simulink model "Snapbot_4_leg"  (R2019b)
settings: Solver=FixedStepAuto  StartTime=0.0  StopTime=10  FixedStep=0.001  RelTol=1e-3
PreLoadFcn:
  | startup_Contact_Forces;
InitFcn:
  | SnapbotParameters;
StopFcn:
  | plot3(out.simout.data(:,1),out.simout.data(:,2),out.simout.data(:,3))
  | hold on;
  | plot3(out.simout.data(:,4),out.simout.data(:,5),out.simout.data(:,6))
  | plot3(out.simout.data(:,7),out.simout.data(:,8),out.simout.data(:,9))
  | plot3(out.simout.data(:,10),out.simout.data(:,11),out.simout.data(:,12))
  | grid on
  | grid minor
  | axis square
  | 
  | view(2)
model workspace (MATLAB code in the model file):
  | % Simscape(TM) Multibody(TM) version: 7.0
  | 
  | % This is a model data file derived from a Simscape Multibody Import XML file using the smimport function.
  | % The data in this file sets the block parameter values in an imported Simscape Multibody model.
  | % For more information on this file, see the smimport function help page in the Simscape Multibody documentation.
  | % You can modify numerical values, but avoid any other changes to this file.
  | % Do not add code to this file. Do not edit the physical units shown in comments.
  | 
  | %%%VariableName:smiData
  | 
  | 
  | %============= RigidTransform =============%
  | 
  | %Initialize the RigidTransform structure array by filling in null values.
  | smiData.RigidTransform(34).translation = [0.0 0.0 0.0];
  | smiData.RigidTransform(34).angle = 0.0;
  | smiData.RigidTransform(34).axis = [0.0 0.0 0.0];
  | smiData.RigidTransform(34).ID = '';
  | 
  | %Translation Method - Cartesian
  | %Rotation Method - Arbitrary Axis
  | smiData.RigidTransform(1).translation = [0 0 3.5000000000000031];  % mm
  | smiData.RigidTransform(1).angle = 0;  % rad
  | smiData.RigidTransform(1).axis = [0 0 0];
  | smiData.RigidTransform(1).ID = 'B[Leg_Assembly_Y-P:Leg_part_01_yaw-1:-:Leg_Assembly_Y-P:v4_Hyb_X-430_IDLE_uncut-1]';
  | 
  | %Translation Method - Cartesian
  | %Rotation Method - Arbitrary Axis
  | smiData.RigidTransform(2).translation = [-1.7352785874891197e-13 -35.250000000000064 1.6342482922482304e-13];  % mm
  | smiData.RigidTransform(2).angle = 3.1415926535897931;  % rad
  | smiData.RigidTransform(2).axis = [0 0.70710678118654746 0.70710678118654757];
  | smiData.RigidTransform(2).ID = 'F[Leg_Assembly_Y-P:Leg_part_01_yaw-1:-:Leg_Assembly_Y-P:v4_Hyb_X-430_IDLE_uncut-1]';
  | 
  | %Translation Method - Cartesian
  | %Rotation Method - Arbitrary Axis
  | smiData.RigidTransform(3).translation = [18.999999999999989 0 -21.500000000000018];  % mm
  | smiData.RigidTransform(3).angle = 2.0943951023931957;  % rad
  | smiData.RigidTransform(3).axis = [0.57735026918962562 0.57735026918962584 0.57735026918962584];
  | smiData.RigidTransform(3).ID = 'B[Leg_Assembly_Y-P:Leg_part_02_Yaw-1:-:Leg_Assembly_Y-P:v4_Hyb_X-430_IDLE_uncut-1]';
  | 
  | %Translation Method - Cartesian
  | %Rotation Method - Arbitrary Axis
  | smiData.RigidTransform(4).translation = [-1.5265566588595902e-12 -1.2221335055073723e-12 19.000000000000597];  % mm
  | smiData.RigidTransform(4).angle = 4.7102773760513257e-16;  % rad
  | smiData.RigidTransform(4).axis = [7.8504622934188734e-17 1 1.8488927466117461e-32];
  | smiData.RigidTransform(4).ID = 'F[Leg_Assembly_Y-P:Leg_part_02_Yaw-1:-:Leg_Assembly_Y-P:v4_Hyb_X-430_IDLE_uncut-1]';
  | 
  | %Translation Method - Cartesian
  | %Rotation Method - Arbitrary Axis
  | smiData.RigidTransform(5).translation = [8.3000000000000025 6 -1.5000000000000013];  % mm
  | smiData.RigidTransform(5).angle = 3.1415926535897931;  % rad
  | smiData.RigidTransform(5).axis = [1 0 0];
  | smiData.RigidTransform(5).ID = 'B[Leg_Assembly_Y-P:Leg_part_02_Yaw-1:-:Leg_Assembly_Y-P:v4_Hyb_X-430_IDLE_uncut-2]';
  | 
  | %Translation Method - Cartesian
  | %Rotation Method - Arbitrary Axis
  | smiData.RigidTransform(6).translation = [-8.0000000000000178 -36.75000000000005 6.0000000000000284];  % mm
  | smiData.RigidTransform(6).angle = 3.1415926535897931;  % rad
  | smiData.RigidTransform(6).axis = [-0 0.70710678118654757 -0.70710678118654746];
  | smiData.RigidTransform(6).ID = 'F[Leg_Assembly_Y-P:Leg_part_02_Yaw-1:-:Leg_Assembly_Y-P:v4_Hyb_X-430_IDLE_uncut-2]';
  | 
  | %Translation Method - Cartesian
  | %Rotation Method - Arbitrary Axis
  | smiData.RigidTransform(7).translation = [-5.7500000000000053 17.750000000000004 20.999999999999993];  % mm
  | smiData.RigidTransform(7).angle = 2.0943951023931953;  % rad
  | smiData.RigidTransform(7).axis = [0.57735026918962584 -0.57735026918962584 0.57735026918962584];
  | smiData.RigidTransform(7).ID = 'B[Leg_Assembly_Y-P:Leg_part_03-1:-:Leg_Assembly_Y-P:v4_Hyb_X-430_IDLE_uncut-2]';
  | 
  | %Translation Method - Cartesian
  | %Rotation Method - Arbitrary Axis
  | smiData.RigidTransform(8).translation = [-17.749999999998572 -3.9999999999999183 5.9999999999999556];  % mm
  | smiData.RigidTransform(8).angle = 2.0943951023931953;  % rad
  | smiData.RigidTransform(8).axis = [0.57735026918962584 0.57735026918962584 0.57735026918962584];
  | smiData.RigidTransform(8).ID = 'F[Leg_Assembly_Y-P:Leg_part_03-1:-:Leg_Assembly_Y-P:v4_Hyb_X-430_IDLE_uncut-2]';
  | 
  | %Translation Method - Cartesian
  | %Rotation Method - Arbitrary Axis
  | smiData.RigidTransform(9).translation = [48 0 0];  % mm
  | smiData.RigidTransform(9).angle = 2.0943951023931953;  % rad
  | smiData.RigidTransform(9).axis = [-0.57735026918962584 -0.57735026918962584 0.57735026918962584];
  | smiData.RigidTransform(9).ID = 'B[Leg_Assembly_Y-P:Leg_part_04-1:-:Leg_Assembly_Y-P:v4_Hyb_X-430_IDLE_uncut-2]';
  | 
  | %Translation Method - Cartesian
  | %Rotation Method - Arbitrary Axis
  | smiData.RigidTransform(10).translation = [-1.8746248997558723e-10 -7.7324813219092903e-12 24.00000000000599];  % mm
  | smiData.RigidTransform(10).angle = 3.1415926535897927;  % rad
  | smiData.RigidTransform(10).axis = [-1 -5.392603844284259e-33 2.7755575615628907e-17];
  | smiData.RigidTransform(10).ID = 'F[Leg_Assembly_Y-P:Leg_part_04-1:-:Leg_Assembly_Y-P:v4_Hyb_X-430_IDLE_uncut-2]';
  | 
  | %Translation Method - Cartesian
  | %Rotation Method - Arbitrary Axis
  | smiData.RigidTransform(11).translation = [21.999999999999993 6.0000000000000124 -15.000000000000009];  % mm
  | smiData.RigidTransform(11).angle = 0;  % rad
  | smiData.RigidTransform(11).axis = [0 0 0];
  | smiData.RigidTransform(11).ID = 'B[Leg_Assembly_Y-P:Leg_part_03-1:-:Leg_Assembly_Y-P:Leg_part_06-1]';
  | 
  | %Translation Method - Cartesian
  | %Rotation Method - Arbitrary Axis
  | smiData.RigidTransform(12).translation = [-25.499999999999105 -3.2214586553891422e-10 -47.43000000032751];  % mm
  | smiData.RigidTransform(12).angle = 2.0943951023931828;  % rad
  | smiData.RigidTransform(12).axis = [0.5773502691896234 0.57735026918962151 0.57735026918963239];
  | smiData.RigidTransform(12).ID = 'F[Leg_Assembly_Y-P:Leg_part_03-1:-:Leg_Assembly_Y-P:Leg_part_06-1]';
  | 
  | %Translation Method - Cartesian
  | %Rotation Method - Arbitrary Axis
  | smiData.RigidTransform(13).translation = [18.500000000000004 0 0];  % mm
  | smiData.RigidTransform(13).angle = 2.0943951023931957;  % rad
  | smiData.RigidTransform(13).axis = [-0.57735026918962584 -0.57735026918962573 0.57735026918962573];
  | smiData.RigidTransform(13).ID = 'B[Leg_Assembly_Y-P:Leg_part_05-1:-:Leg_Assembly_Y-P:Leg_part_04-1]';
  | 
  | %Translation Method - Cartesian
  | %Rotation Method - Arbitrary Axis
  | smiData.RigidTransform(14).translation = [5.4999999999949978 -8.3794303905713249e-10 -60.000000000037232];  % mm
  | smiData.RigidTransform(14).angle = 2.0943951023931917;  % rad
  | smiData.RigidTransform(14).axis = [0.57735026918961896 0.57735026918962451 0.57735026918963384];
  | smiData.RigidTransform(14).ID = 'F[Leg_Assembly_Y-P:Leg_part_05-1:-:Leg_Assembly_Y-P:Leg_part_04-1]';
  | 
  | %Translation Method - Cartesian
  | %Rotation Method - Arbitrary Axis
  | smiData.RigidTransform(15).translation = [-4.5000000000000009 25.000000000000004 0];  % mm
  | smiData.RigidTransform(15).angle = 2.0943951023931953;  % rad
  | smiData.RigidTransform(15).axis = [-0.57735026918962584 -0.57735026918962584 0.57735026918962584];
  | smiData.RigidTransform(15).ID = 'B[Leg_Assembly_Y-P:Leg_part_05-1:-:Leg_Assembly_Y-P:Leg_part_06-1]';
  | 
  | %Translation Method - Cartesian
  | %Rotation Method - Arbitrary Axis
  | smiData.RigidTransform(16).translation = [9.0000000000012914 1.0276604186564152e-10 7.8563660354995227e-11];  % mm
  | smiData.RigidTransform(16).angle = 2.0943951023931957;  % rad
  | smiData.RigidTransform(16).axis = [0.57735026918962573 0.57735026918962595 0.57735026918962562];
  | smiData.RigidTransform(16).ID = 'F[Leg_Assembly_Y-P:Leg_part_05-1:-:Leg_Assembly_Y-P:Leg_part_06-1]';
  | 
  | %Translation Method - Cartesian
  | %Rotation Method - Arbitrary Axis
  | smiData.RigidTransform(17).translation = [-29.148138792437695 31.324765133364561 -50.486057334570788];  % mm
  | smiData.RigidTransform(17).angle = 0.85969556486762955;  % rad
  | smiData.RigidTransform(17).axis = [-0.88342402684813537 0.43430848851138693 -0.17589236934665334];
  | smiData.RigidTransform(17).ID = 'B[Body_Frame-2:-:cover_IMU-1]';
  | 
  | %Translation Method - Cartesian
  | %Rotation Method - Arbitrary Axis
  | smiData.RigidTransform(18).translation = [-29.14813879243771 -3.6752348666354493 -50.486057334570788];  % mm
  | smiData.RigidTransform(18).angle = 0.85969556486762955;  % rad
  | smiData.RigidTransform(18).axis = [-0.88342402684813537 0.43430848851138693 -0.17589236934665334];
  | smiData.RigidTransform(18).ID = 'F[Body_Frame-2:-:cover_IMU-1]';
  | 
  | %Translation Method - Cartesian
  | %Rotation Method - Arbitrary Axis
  | smiData.RigidTransform(19).translation = [-17.98437038909324 16.010419740604625 -58.898751217406286];  % mm
  | smiData.RigidTransform(19).angle = 2.5668813081404753;  % rad
  | smiData.RigidTransform(19).axis = [-0.54469904781872214 -0.67552162020226258 0.49696427230203144];
  | smiData.RigidTransform(19).ID = 'B[Body_Frame-2:-:Leg_Assembly_Y-P-4:Leg_part_01_yaw-1]';
  | 
  | %Translation Method - Cartesian
  | %Rotation Method - Arbitrary Axis
  | smiData.RigidTransform(20).translation = [-13.874453980679554 8.010419740604668 -21.000000000000121];  % mm
  | smiData.RigidTransform(20).angle = 1.5933089052267591;  % rad
  | smiData.RigidTransform(20).axis = [0.454741574326607 0.14837486987204307 0.87817708838787945];
  | smiData.RigidTransform(20).ID = 'F[Body_Frame-2:-:Leg_Assembly_Y-P-4:Leg_part_01_yaw-1]';
  | 
  | %Translation Method - Cartesian
  | %Rotation Method - Arbitrary Axis
  | smiData.RigidTransform(21).translation = [29.999999999999968 24.020839481209347 -51.961524227066349];  % mm
  | smiData.RigidTransform(21).angle = 2.3875525638501713;  % rad
  | smiData.RigidTransform(21).axis = [0.97769691900991618 0.078837114487629617 0.19466238449629056];
  | smiData.RigidTransform(21).ID = 'B[Body_Frame-2:-:Leg_Assembly_Y-P-3:Leg_part_01_yaw-1]';
  | 
  | %Translation Method - Cartesian
  | %Rotation Method - Arbitrary Axis
  | smiData.RigidTransform(22).translation = [-2.6467716907063732e-13 16.020839481209734 -21.000000000000327];  % mm
  | smiData.RigidTransform(22).angle = 2.8078721686781996;  % rad
  | smiData.RigidTransform(22).axis = [0.061302152168851563 -0.3413768904692025 0.9379252980877768];
  | smiData.RigidTransform(22).ID = 'F[Body_Frame-2:-:Leg_Assembly_Y-P-3:Leg_part_01_yaw-1]';
  | 
  | %Translation Method - Cartesian
  | %Rotation Method - Arbitrary Axis
  | smiData.RigidTransform(23).translation = [30.000000000000529 24.020839481209347 51.961524227066029];  % mm
  | smiData.RigidTransform(23).angle = 0.85969556486763532;  % rad
  | smiData.RigidTransform(23).axis = [0.88342402684813182 0.43430848851139281 0.17589236934665636];
  | smiData.RigidTransform(23).ID = 'B[Body_Frame-2:-:Leg_Assembly_Y-P-2:Leg_part_01_yaw-1]';
  | 
  | %Translation Method - Cartesian
  | %Rotation Method - Arbitrary Axis
  | smiData.RigidTransform(24).translation = [3.3395508580724709e-13 16.020839481209283 -21.000000000000096];  % mm
  | smiData.RigidTransform(24).angle = 0.78005530127659528;  % rad
  | smiData.RigidTransform(24).axis = [0.88538441591606198 -0.1589913427291928 0.43682512403723089];
  | smiData.RigidTransform(24).ID = 'F[Body_Frame-2:-:Leg_Assembly_Y-P-2:Leg_part_01_yaw-1]';
  | 
  | %Translation Method - Cartesian
  | %Rotation Method - Arbitrary Axis
  | smiData.RigidTransform(25).translation = [0 16.0208394812094 -21.000000000000004];  % mm
  | smiData.RigidTransform(25).angle = 2.4434609527920594;  % rad
  | smiData.RigidTransform(25).axis = [-1 -2.4245288061633076e-16 6.6613381477509383e-16];
  | smiData.RigidTransform(25).ID = 'B[Leg_Assembly_Y-P-1:Leg_part_01_yaw-1:-:Body_Frame-2]';
  | 
  | %Translation Method - Cartesian
  | %Rotation Method - Arbitrary Axis
  | smiData.RigidTransform(26).translation = [-29.999999999999616 24.020839481209507 51.961524227066668];  % mm
  | smiData.RigidTransform(26).angle = 2.4682098215588222;  % rad
  | smiData.RigidTransform(26).axis = [-0.96166828182989783 -0.093787209197190524 -0.25767823950294055];
  | smiData.RigidTransform(26).ID = 'F[Leg_Assembly_Y-P-1:Leg_part_01_yaw-1:-:Body_Frame-2]';
  | 
  | %Translation Method - Cartesian
  | %Rotation Method - Arbitrary Axis
  | smiData.RigidTransform(27).translation = [58.296277584874822 -3.6752348666354502 0];  % mm
  | smiData.RigidTransform(27).angle = 1.750366012803156;  % rad
  | smiData.RigidTransform(27).axis = [0.83481712947898612 0.38928162063502708 0.38928162063502636];
  | smiData.RigidTransform(27).ID = 'B[cover-2:-:Body_Frame-2]';
  | 
  | %Translation Method - Cartesian
  | %Rotation Method - Arbitrary Axis
  | smiData.RigidTransform(28).translation = [-58.29627758487473 -15.324765133364487 1.1215639593173864e-12];  % mm
  | smiData.RigidTransform(28).angle = 2.5346467848844099;  % rad
  | smiData.RigidTransform(28).axis = [0.31314561301496879 -0.67154293423781619 -0.67154293423782185];
  | smiData.RigidTransform(28).ID = 'F[cover-2:-:Body_Frame-2]';
  | 
  | %Translation Method - Cartesian
  | %Rotation Method - Arbitrary Axis
  | smiData.RigidTransform(29).translation = [-0.53570167355018738 37.318511693782625 54.569829435763872];  % mm
  | smiData.RigidTransform(29).angle = 0;  % rad
  | smiData.RigidTransform(29).axis = [0 0 0];
  | smiData.RigidTransform(29).ID = 'AssemblyGround[Leg_Assembly_Y-P-1:Leg_part_01_yaw-1]';
  | 
  | %Translation Method - Cartesian
  | %Rotation Method - Arbitrary Axis
  | smiData.RigidTransform(30).translation = [-0.53570167355018394 37.318511693782625 54.569829435763872];  % mm
  | smiData.RigidTransform(30).angle = 0;  % rad
  | smiData.RigidTransform(30).axis = [0 0 0];
  | smiData.RigidTransform(30).ID = 'AssemblyGround[Leg_Assembly_Y-P-3:Leg_part_01_yaw-1]';
  | 
  | %Translation Method - Cartesian
  | %Rotation Method - Arbitrary Axis
  | smiData.RigidTransform(31).translation = [-0.53570167355018217 37.318511693782625 54.56982943576385];  % mm
  | smiData.RigidTransform(31).angle = 0;  % rad
  | smiData.RigidTransform(31).axis = [0 0 0];
  | smiData.RigidTransform(31).ID = 'AssemblyGround[Leg_Assembly_Y-P-4:Leg_part_01_yaw-1]';
  | 
  | %Translation Method - Cartesian
  | %Rotation Method - Arbitrary Axis
  | smiData.RigidTransform(32).translation = [-0.53570167355018561 37.318511693782625 54.569829435763886];  % mm
  | smiData.RigidTransform(32).angle = 0;  % rad
  | smiData.RigidTransform(32).axis = [0 0 0];
  | smiData.RigidTransform(32).ID = 'AssemblyGround[Leg_Assembly_Y-P-2:Leg_part_01_yaw-1]';
  | 
  | %Translation Method - Cartesian
  | %Rotation Method - Arbitrary Axis
  | smiData.RigidTransform(33).translation = [16.947427364988048 -132.5 -0.35447398452139084];  % mm
  | smiData.RigidTransform(33).angle = 0;  % rad
  | smiData.RigidTransform(33).axis = [0 0 0];
  | smiData.RigidTransform(33).ID = 'RootGround[floor-1]';
  | 
  | %Translation Method - Cartesian
  | %Rotation Method - Arbitrary Axis
  | smiData.RigidTransform(34).translation = [2.4083582801206584 -17.449369734884318 -0.97062236223489184];  % mm
  | smiData.RigidTransform(34).angle = 3.1415926535897927;  % rad
  | smiData.RigidTransform(34).axis = [-1.8561360843499775e-09 2.3245294513264802e-16 1];
  | smiData.RigidTransform(34).ID = 'SixDofRigidTransform[cover-2]';
  | 
  | 
  | %============= Solid =============%
  | %Center of Mass (CoM) %Moments of Inertia (MoI) %Product of Inertia (PoI)
  | 
  | %Initialize the Solid structure array by filling in null values.
  | smiData.Solid(11).mass = 0.0;
  | smiData.Solid(11).CoM = [0.0 0.0 0.0];
  | smiData.Solid(11).MoI = [0.0 0.0 0.0];
  | smiData.Solid(11).PoI = [0.0 0.0 0.0];
  | smiData.Solid(11).color = [0.0 0.0 0.0];
  | smiData.Solid(11).opacity = 0.0;
  | smiData.Solid(11).ID = '';
  | 
  | %Inertia Type - Custom
  | %Visual Properties - Simple
  | smiData.Solid(1).mass = 0.011859040673008397;  % kg
  | smiData.Solid(1).CoM = [9.2568952005630604e-05 1.191765890643393 -6.4265217754949023e-05];  % mm
  | smiData.Solid(1).MoI = [12.336903139260382 24.543407766477525 12.336924066027152];  % kg*mm^2
  | smiData.Solid(1).PoI = [1.0093449377553896e-06 3.0788090295607977e-05 -1.064469578641841e-06];  % kg*mm^2
  | smiData.Solid(1).color = [0.792156862745098 0.81960784313725488 0.93333333333333335];
  | smiData.Solid(1).opacity = 1;
  | smiData.Solid(1).ID = 'cover*:*Default';
  | 
  | %Inertia Type - Custom
  | %Visual Properties - Simple
  | smiData.Solid(2).mass = 0.012023631787858334;  % kg
  | smiData.Solid(2).CoM = [-0.29734349259876186 1.2054189328895923 0.00017861160100909334];  % mm
  | smiData.Solid(2).MoI = [12.313344376366921 24.562977425030333 12.378785765398183];  % kg*mm^2
  | smiData.Solid(2).PoI = [1.0647394470527272e-05 -8.7602005901832794e-05 0.00062815776109033676];  % kg*mm^2
  | smiData.Solid(2).color = [0.792156862745098 0.81960784313725488 0.93333333333333335];
  | smiData.Solid(2).opacity = 1;
  | smiData.Solid(2).ID = 'cover_IMU*:*Default';
  | 
  | %Inertia Type - Custom
  | %Visual Properties - Simple
  | smiData.Solid(3).mass = 0.01532092516699415;  % kg
  | smiData.Solid(3).CoM = [23.99999768920209 1.296167806282416 -35.100094443023529];  % mm
  | smiData.Solid(3).MoI = [10.22123294031608 14.203511884952171 5.0157635391797406];  % kg*mm^2
  | smiData.Solid(3).PoI = [0.58071119483444822 9.2473756106630214e-07 -5.4914041407852197e-06];  % kg*mm^2
  | smiData.Solid(3).color = [1 0.38823529411764707 0.41960784313725491];
  | smiData.Solid(3).opacity = 1;
  | smiData.Solid(3).ID = 'Leg_part_04*:*Default';
  | 
  | %Inertia Type - Custom
  | %Visual Properties - Simple
  | smiData.Solid(4).mass = 0.022715083434313929;  % kg
  | smiData.Solid(4).CoM = [4.7495790017590746e-05 -5.291488289899466e-07 0.51650579217012571];  % mm
  | smiData.Solid(4).MoI = [6.0201227624572118 7.3567997591054697 10.813457729002581];  % kg*mm^2
  | smiData.Solid(4).PoI = [5.9445977678909571e-08 -2.8721317733849146e-06 -2.6844578170485016e-06];  % kg*mm^2
  | smiData.Solid(4).color = [0.027450980392156862 1 0.027450980392156862];
  | smiData.Solid(4).opacity = 1;
  | smiData.Solid(4).ID = 'Leg_part_02_Yaw*:*Default';
  | 
  | %Inertia Type - Custom
  | %Visual Properties - Simple
  | smiData.Solid(5).mass = 0.0061788723822202912;  % kg
  | smiData.Solid(5).CoM = [4.2543802409912486 -4.6300920972242539 -20.149819352752832];  % mm
  | smiData.Solid(5).MoI = [2.2893274182864185 2.0053458866812135 0.35993641872183124];  % kg*mm^2
  | smiData.Solid(5).PoI = [0.20173149787382891 -0.0054107076234519375 0.0070268738351532264];  % kg*mm^2
  | smiData.Solid(5).color = [0.8666666666666667 0.46666666666666667 0.094117647058823528];
  | smiData.Solid(5).opacity = 1;
  | smiData.Solid(5).ID = 'Leg_part_06*:*Default';
  | 
  | %Inertia Type - Custom
  | %Visual Properties - Simple
  | smiData.Solid(6).mass = 0.022008322051922567;  % kg
  | smiData.Solid(6).CoM = [-0.00020078562164607593 -0.086645709821882896 -7.0226871847428294];  % mm
  | smiData.Solid(6).MoI = [6.5441760223709844 5.812065440337185 5.5882327823375331];  % kg*mm^2
  | smiData.Solid(6).PoI = [-0.022603449848343178 -3.3526868327938216e-05 -5.8881839764321484e-05];  % kg*mm^2
  | smiData.Solid(6).color = [0.9882352941176471 0.73725490196078436 0.51764705882352935];
  | smiData.Solid(6).opacity = 1;
  | smiData.Solid(6).ID = 'Leg_part_01_yaw*:*Default';
  | 
  | %Inertia Type - Custom
  | %Visual Properties - Simple
  | smiData.Solid(7).mass = 0.015928924279537775;  % kg
  | smiData.Solid(7).CoM = [5.5724533955433548 0.60923661115773253 14.965495324586268];  % mm
  | smiData.Solid(7).MoI = [6.7178267454302487 3.3961346093070595 5.3516535264104625];  % kg*mm^2
  | smiData.Solid(7).PoI = [0.0029589860947701109 0.0090414356066351384 -0.14024072638650095];  % kg*mm^2
  | smiData.Solid(7).color = [0.50196078431372548 1 1];
  | smiData.Solid(7).opacity = 1;
  | smiData.Solid(7).ID = 'Leg_part_03*:*Default';
  | 
  | %Inertia Type - Custom
  | %Visual Properties - Simple
  | smiData.Solid(8).mass = 0.014765646142892601;  % kg
  | smiData.Solid(8).CoM = [1.2086758180566385e-05 38.516029865216893 1.6102137949923504e-05];  % mm
  | smiData.Solid(8).MoI = [11.438112427079185 0.88080259805912409 11.92628093115035];  % kg*mm^2
  | smiData.Solid(8).PoI = [1.3310978325613474e-06 5.7966270338224739e-06 1.0118234092923484e-06];  % kg*mm^2
  | smiData.Solid(8).color = [0.039215686274509803 0.63137254901960782 0.90588235294117647];
  | smiData.Solid(8).opacity = 1;
  | smiData.Solid(8).ID = 'Leg_part_05*:*Default';
  | 
  | %Inertia Type - Custom
  | %Visual Properties - Simple
  | smiData.Solid(9).mass = 0.043283962506312147;  % kg
  | smiData.Solid(9).CoM = [0 -11.629154441205351 0.58622657822569424];  % mm
  | smiData.Solid(9).MoI = [11.945660403890638 6.9373449472329343 10.473897647404554];  % kg*mm^2
  | smiData.Solid(9).PoI = [-0.010479195470367004 0 0];  % kg*mm^2
  | smiData.Solid(9).color = [0.50196078431372548 0.50196078431372548 0.50196078431372548];
  | smiData.Solid(9).opacity = 1;
  | smiData.Solid(9).ID = 'v4_Hyb_X-430_IDLE_uncut*:*Default';
  | 
  | %Inertia Type - Custom
  | %Visual Properties - Simple
  | smiData.Solid(10).mass = 0.06914285683427808;  % kg
  | smiData.Solid(10).CoM = [-6.5363881170266666e-08 8.0286872966298493 -0.84505300940729655];  % mm
  | smiData.Solid(10).MoI = [133.83817269769423 248.31514966138266 134.30804068565411];  % kg*mm^2
  | smiData.Solid(10).PoI = [0.10611953301327913 3.6362610588971529e-07 -3.5551675916145607e-07];  % kg*mm^2
  | smiData.Solid(10).color = [0.75294117647058822 0.75294117647058822 0.75294117647058822];
  | smiData.Solid(10).opacity = 1;
  | smiData.Solid(10).ID = 'Body_Frame*:*Default';
  | 
  | %Inertia Type - Custom
  | %Visual Properties - Simple
  | smiData.Solid(11).mass = 49.999999999999993;  % kg
  | smiData.Solid(11).CoM = [0 25.000000000000004 0];  % mm
  | smiData.Solid(11).MoI = [4177083.333333334 8333333.3333333358 4177083.333333333];  % kg*mm^2
  | smiData.Solid(11).PoI = [0 -7.6327832942979522e-10 0];  % kg*mm^2
  | smiData.Solid(11).color = [0.792156862745098 0.81960784313725488 0.93333333333333335];
  | smiData.Solid(11).opacity = 1;
  | smiData.Solid(11).ID = 'floor*:*Default';
  | 
  | 
  | %============= Joint =============%
  | %X Revolute Primitive (Rx) %Y Revolute Primitive (Ry) %Z Revolute Primitive (Rz)
  | %X Prismatic Primitive (Px) %Y Prismatic Primitive (Py) %Z Prismatic Primitive (Pz) %Spherical Primitive (S)
  | %Constant Velocity Primitive (CV) %Lead Screw Primitive (LS)
  | %Position Target (Pos)
  | 
  | %Initialize the CylindricalJoint structure array by filling in null values.
  | smiData.CylindricalJoint(4).Rz.Pos = 0.0;
  | smiData.CylindricalJoint(4).Pz.Pos = 0.0;
  | smiData.CylindricalJoint(4).ID = '';
  | 
  | %This joint has been chosen as a cut joint. Simscape Multibody treats cut joints as algebraic constraints to solve closed kinematic loops. The imported model does not use the state target data for this joint.
  | smiData.CylindricalJoint(1).Rz.Pos = -40.005411760834875;  % deg
  | smiData.CylindricalJoint(1).Pz.Pos = 0;  % mm
  | smiData.CylindricalJoint(1).ID = '[Leg_Assembly_Y-P-1:Leg_part_05-1:-:Leg_Assembly_Y-P-1:Leg_part_06-1]';
  | 
  | %This joint has been chosen as a cut joint. Simscape Multibody treats cut joints as algebraic constraints to solve closed kinematic loops. The imported model does not use the state target data for this joint.
  | smiData.CylindricalJoint(2).Rz.Pos = -40.005411760841149;  % deg
  | smiData.CylindricalJoint(2).Pz.Pos = 0;  % mm
  | smiData.CylindricalJoint(2).ID = '[Leg_Assembly_Y-P-3:Leg_part_05-1:-:Leg_Assembly_Y-P-3:Leg_part_06-1]';
  | 
  | %This joint has been chosen as a cut joint. Simscape Multibody treats cut joints as algebraic constraints to solve closed kinematic loops. The imported model does not use the state target data for this joint.
  | smiData.CylindricalJoint(3).Rz.Pos = -40.005411760676694;  % deg
  | smiData.CylindricalJoint(3).Pz.Pos = 0;  % mm
  | smiData.CylindricalJoint(3).ID = '[Leg_Assembly_Y-P-4:Leg_part_05-1:-:Leg_Assembly_Y-P-4:Leg_part_06-1]';
  | 
  | %This joint has been chosen as a cut joint. Simscape Multibody treats cut joints as algebraic constraints to solve closed kinematic loops. The imported model does not use the state target data for this joint.
  | smiData.CylindricalJoint(4).Rz.Pos = -40.00541176081142;  % deg
  | smiData.CylindricalJoint(4).Pz.Pos = 0;  % mm
  | smiData.CylindricalJoint(4).ID = '[Leg_Assembly_Y-P-2:Leg_part_05-1:-:Leg_Assembly_Y-P-2:Leg_part_06-1]';
  | 
  | 
  | %Initialize the RevoluteJoint structure array by filling in null values.
  | smiData.RevoluteJoint(20).Rz.Pos = 0.0;
  | smiData.RevoluteJoint(20).ID = '';
  | 
  | smiData.RevoluteJoint(1).Rz.Pos = 8.9959671327898853e-15;  % deg
  | smiData.RevoluteJoint(1).ID = '[Leg_Assembly_Y-P-1:Leg_part_02_Yaw-1:-:Leg_Assembly_Y-P-1:v4_Hyb_X-430_IDLE_uncut-1]';
  | 
  | smiData.RevoluteJoint(2).Rz.Pos = -90;  % deg
  | smiData.RevoluteJoint(2).ID = '[Leg_Assembly_Y-P-1:Leg_part_03-1:-:Leg_Assembly_Y-P-1:v4_Hyb_X-430_IDLE_uncut-2]';
  | 
  | smiData.RevoluteJoint(3).Rz.Pos = 180;  % deg
  | smiData.RevoluteJoint(3).ID = '[Leg_Assembly_Y-P-1:Leg_part_04-1:-:Leg_Assembly_Y-P-1:v4_Hyb_X-430_IDLE_uncut-2]';
  | 
  | smiData.RevoluteJoint(4).Rz.Pos = -130.80925683646444;  % deg
  | smiData.RevoluteJoint(4).ID = '[Leg_Assembly_Y-P-1:Leg_part_03-1:-:Leg_Assembly_Y-P-1:Leg_part_06-1]';
  | 
  | smiData.RevoluteJoint(5).Rz.Pos = -179.19615492437049;  % deg
  | smiData.RevoluteJoint(5).ID = '[Leg_Assembly_Y-P-1:Leg_part_05-1:-:Leg_Assembly_Y-P-1:Leg_part_04-1]';
  | 
  | smiData.RevoluteJoint(6).Rz.Pos = 9.6985521658607794e-11;  % deg
  | smiData.RevoluteJoint(6).ID = '[Leg_Assembly_Y-P-3:Leg_part_02_Yaw-1:-:Leg_Assembly_Y-P-3:v4_Hyb_X-430_IDLE_uncut-1]';
  | 
  | smiData.RevoluteJoint(7).Rz.Pos = -90.000000000000014;  % deg
  | smiData.RevoluteJoint(7).ID = '[Leg_Assembly_Y-P-3:Leg_part_03-1:-:Leg_Assembly_Y-P-3:v4_Hyb_X-430_IDLE_uncut-2]';
  | 
  | smiData.RevoluteJoint(8).Rz.Pos = -179.99999999998752;  % deg
  | smiData.RevoluteJoint(8).ID = '[Leg_Assembly_Y-P-3:Leg_part_04-1:-:Leg_Assembly_Y-P-3:v4_Hyb_X-430_IDLE_uncut-2]';
  | 
  | smiData.RevoluteJoint(9).Rz.Pos = -130.80925683643747;  % deg
  | smiData.RevoluteJoint(9).ID = '[Leg_Assembly_Y-P-3:Leg_part_03-1:-:Leg_Assembly_Y-P-3:Leg_part_06-1]';
  | 
  | smiData.RevoluteJoint(10).Rz.Pos = -179.19615492439118;  % deg
  | smiData.RevoluteJoint(10).ID = '[Leg_Assembly_Y-P-3:Leg_part_05-1:-:Leg_Assembly_Y-P-3:Leg_part_04-1]';
  | 
  | smiData.RevoluteJoint(11).Rz.Pos = 1.7991934265579774e-14;  % deg
  | smiData.RevoluteJoint(11).ID = '[Leg_Assembly_Y-P-4:Leg_part_02_Yaw-1:-:Leg_Assembly_Y-P-4:v4_Hyb_X-430_IDLE_uncut-1]';
  | 
  | smiData.RevoluteJoint(12).Rz.Pos = -90;  % deg
  | smiData.RevoluteJoint(12).ID = '[Leg_Assembly_Y-P-4:Leg_part_03-1:-:Leg_Assembly_Y-P-4:v4_Hyb_X-430_IDLE_uncut-2]';
  | 
  | smiData.RevoluteJoint(13).Rz.Pos = 179.99999999960033;  % deg
  | smiData.RevoluteJoint(13).ID = '[Leg_Assembly_Y-P-4:Leg_part_04-1:-:Leg_Assembly_Y-P-4:v4_Hyb_X-430_IDLE_uncut-2]';
  | 
  | smiData.RevoluteJoint(14).Rz.Pos = -130.80925683712383;  % deg
  | smiData.RevoluteJoint(14).ID = '[Leg_Assembly_Y-P-4:Leg_part_03-1:-:Leg_Assembly_Y-P-4:Leg_part_06-1]';
  | 
  | smiData.RevoluteJoint(15).Rz.Pos = -179.19615492395255;  % deg
  | smiData.RevoluteJoint(15).ID = '[Leg_Assembly_Y-P-4:Leg_part_05-1:-:Leg_Assembly_Y-P-4:Leg_part_04-1]';
  | 
  | smiData.RevoluteJoint(16).Rz.Pos = 8.9959671327898869e-15;  % deg
  | smiData.RevoluteJoint(16).ID = '[Leg_Assembly_Y-P-2:Leg_part_02_Yaw-1:-:Leg_Assembly_Y-P-2:v4_Hyb_X-430_IDLE_uncut-1]';
  | 
  | smiData.RevoluteJoint(17).Rz.Pos = -90;  % deg
  | smiData.RevoluteJoint(17).ID = '[Leg_Assembly_Y-P-2:Leg_part_03-1:-:Leg_Assembly_Y-P-2:v4_Hyb_X-430_IDLE_uncut-2]';
  | 
  | smiData.RevoluteJoint(18).Rz.Pos = 180;  % deg
  | smiData.RevoluteJoint(18).ID = '[Leg_Assembly_Y-P-2:Leg_part_04-1:-:Leg_Assembly_Y-P-2:v4_Hyb_X-430_IDLE_uncut-2]';
  | 
  | smiData.RevoluteJoint(19).Rz.Pos = -130.80925683656244;  % deg
  | smiData.RevoluteJoint(19).ID = '[Leg_Assembly_Y-P-2:Leg_part_03-1:-:Leg_Assembly_Y-P-2:Leg_part_06-1]';
  | 
  | smiData.RevoluteJoint(20).Rz.Pos = -179.19615492424902;  % deg
  | smiData.RevoluteJoint(20).ID = '[Leg_Assembly_Y-P-2:Leg_part_05-1:-:Leg_Assembly_Y-P-2:Leg_part_04-1]';
values from neighbouring files (symbols this model uses):
  mass_xm430 = 82    [SnapbotParameters.m]
undefined symbols (not defined in the file or in its folder): smiData, X, Y, Z
libraries: sm_lib x191, nesl_utility x28, Contact_Forces_Lib x10
(part 1 of 6)
settings Model: Creator=Kevin_Home  LastModifiedBy=Kevin_Home
settings ExplorerConfigSet: InternalSimMechanicsExplorerSettings="<ExplorerConfiguration><canonicalview>default</canonicalview><AnimationSetting><BasePlaybackSpeed>1.0</BasePlaybackSpeed><PlaybackSpeedFactor>1.0</PlaybackSpeedFactor></AnimationSetting><TilePanel><TileInfo><Tiles Columns=\"1\" Count=\"1\" Rows=\"1\"><Column Weight=\"1\"/><Row Weight=\"1\"/><Tile Height=\"1\" Width=\"1\" X=\"0\" Y=\"0\"/></Tiles></TileInfo><SceneInfo><SceneViewer><BGColor><R>0.60000002384185791</R><G>1</G><B>1</B></BGColor><Camera><DoPerspective>off</DoPerspective><Position><X>-217.246830094688079</X><Y>113.108474411831537</Y><Z>52.8872630286014385</Z></Position><Center><X>-0.902430327962377987</X><Y>0.229218017573074917</Y><Z>0.175732092976339516</Z></Center><Up><X>0.442868139606599265</X><Y>0.8918375727327299</Y><Z>-0.0921604838506315804</Z></Up><ViewLimDist>1</ViewLimDist><YLim>0.501072049732542601</YLim><XLim>0.806169253347468473</XLim></Camera></SceneViewer></SceneInfo></TilePanel><MechEditorPanel><Cameras/><GfxPanelCameraMap/><VideoCreator><PlaybackSpeedRatio>1.0</PlaybackSpeedRatio><FrameRate>30</FrameRate><VideoFormat>MPEG-4</VideoFormat><FrameSize>auto</FrameSize></VideoCreator></MechEditorPanel></ExplorerConfiguration>"

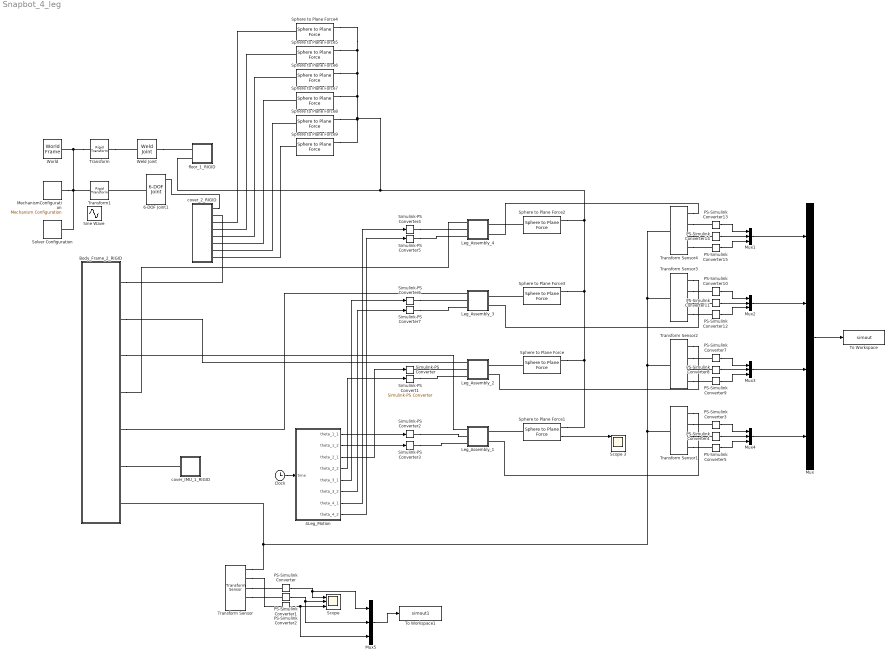
== system Snapbot_4_leg ==
  4Leg_Motion : MATLAB Function  TreatAsAtomicUnit=on
  6-DOF Joint1 : sm_lib/Joints/6-DOF Joint  JointMode=Normal  SenseConstraintForce=off  SenseConstraintForceX=off  SenseConstraintForceY=off  SenseConstraintForceZ=off  SenseConstraintTorque=off  SenseConstraintTorqueX=off  SenseConstraintTorqueY=off  SenseConstraintTorqueZ=off  SenseTotalForce=off  SenseTotalForceX=off  SenseTotalForceY=off  SenseTotalForceZ=off  SenseTotalTorque=off  SenseTotalTorqueX=off  SenseTotalTorqueY=off  SenseTotalTorqueZ=off  CompositeWrenchDir=FollowerOnBase  CompositeWrenchFrame=BaseFrame  PxEquilibriumPosition=0  PxEquilibriumPositionUnits=m  PxSpringStiffness=0  PxSpringStiffnessUnits=N/m  PxDampingCoefficient=0  PxDampingCoefficientUnits=N/(m/s)  PxTorqueActuationMode=NoTorque  PxMotionActuationMode=ComputedMotion  PxSensePosition=on  PxSenseVelocity=off  PxSenseAcceleration=off  PxSenseTorqueForce=off  PxSenseLowerLimitTorqueForce=off  PxSenseUpperLimitTorqueForce=off  PxLowerLimitSpecify=off  PxLowerLimitBound=-1  PxLowerLimitBoundUnits=m  PxLowerLimitStiffness=1e6  PxLowerLimitStiffnessUnits=N/m  PxLowerLimitDamping=1e3  PxLowerLimitDampingUnits=N/(m/s)  PxLowerLimitTransitionRegionWidth=1e-4  PxLowerLimitTransitionRegionWidthUnits=m  PxUpperLimitSpecify=off  PxUpperLimitBound=1  PxUpperLimitBoundUnits=m  PxUpperLimitStiffness=1e6  PxUpperLimitStiffnessUnits=N/m  PxUpperLimitDamping=1e3  PxUpperLimitDampingUnits=N/(m/s)  PxUpperLimitTransitionRegionWidth=1e-4  PxUpperLimitTransitionRegionWidthUnits=m  PxPositionTargetSpecify=off  PxPositionTargetPriority=High  PxPositionTargetValue=0  PxPositionTargetValueUnits=m  PxVelocityTargetSpecify=off  PxVelocityTargetPriority=High  PxVelocityTargetValue=0  PxVelocityTargetValueUnits=m/s  PyEquilibriumPosition=0  PyEquilibriumPositionUnits=m  PySpringStiffness=0  PySpringStiffnessUnits=N/m  PyDampingCoefficient=0  PyDampingCoefficientUnits=N/(m/s)  PyTorqueActuationMode=NoTorque  PyMotionActuationMode=ComputedMotion  PySensePosition=on  PySenseVelocity=off  PySenseAcceleration=off  PySenseTorqueForce=off  PySenseLowerLimitTorqueForce=off  PySenseUpperLimitTorqueForce=off  PyLowerLimitSpecify=off  PyLowerLimitBound=-1  PyLowerLimitBoundUnits=m  PyLowerLimitStiffness=1e6  PyLowerLimitStiffnessUnits=N/m  PyLowerLimitDamping=1e3  PyLowerLimitDampingUnits=N/(m/s)  PyLowerLimitTransitionRegionWidth=1e-4  PyLowerLimitTransitionRegionWidthUnits=m  PyUpperLimitSpecify=off  PyUpperLimitBound=1  PyUpperLimitBoundUnits=m  PyUpperLimitStiffness=1e6  PyUpperLimitStiffnessUnits=N/m  PyUpperLimitDamping=1e3  PyUpperLimitDampingUnits=N/(m/s)  PyUpperLimitTransitionRegionWidth=1e-4  PyUpperLimitTransitionRegionWidthUnits=m  PyPositionTargetSpecify=off  PyPositionTargetPriority=High  PyPositionTargetValue=0  PyPositionTargetValueUnits=m  PyVelocityTargetSpecify=off  PyVelocityTargetPriority=High  PyVelocityTargetValue=0  PyVelocityTargetValueUnits=m/s  PzEquilibriumPosition=0  PzEquilibriumPositionUnits=m  PzSpringStiffness=0  PzSpringStiffnessUnits=N/m  PzDampingCoefficient=0  PzDampingCoefficientUnits=N/(m/s)  PzTorqueActuationMode=NoTorque  PzMotionActuationMode=ComputedMotion  PzSensePosition=on  PzSenseVelocity=off  PzSenseAcceleration=off  PzSenseTorqueForce=off  PzSenseLowerLimitTorqueForce=off  PzSenseUpperLimitTorqueForce=off  PzLowerLimitSpecify=off  PzLowerLimitBound=-1  PzLowerLimitBoundUnits=m  PzLowerLimitStiffness=1e6  PzLowerLimitStiffnessUnits=N/m  PzLowerLimitDamping=1e3  PzLowerLimitDampingUnits=N/(m/s)  PzLowerLimitTransitionRegionWidth=1e-4  PzLowerLimitTransitionRegionWidthUnits=m  PzUpperLimitSpecify=off  PzUpperLimitBound=1  PzUpperLimitBoundUnits=m  PzUpperLimitStiffness=1e6  PzUpperLimitStiffnessUnits=N/m  PzUpperLimitDamping=1e3  PzUpperLimitDampingUnits=N/(m/s)  PzUpperLimitTransitionRegionWidth=1e-4  PzUpperLimitTransitionRegionWidthUnits=m  PzPositionTargetSpecify=off  PzPositionTargetPriority=High  PzPositionTargetValue=0  PzPositionTargetValueUnits=m  PzVelocityTargetSpecify=off  PzVelocityTargetPriority=High  PzVelocityTargetValue=0  PzVelocityTargetValueUnits=m/s  SphDefPosRotationMethod=None  SphDefPosRotationAngleUnits=deg  SphDefPosRotationStandardAxis=+Z  SphDefPosRotationAngle=0.0  SphDefPosRotationArbitraryAxis=[0 0 1]  SphDefPosFollAlignAxisA=+X  SphDefPosBaseAlignAxisA=+Y  SphDefPosFollAlignAxisB=+Y  SphDefPosBaseAlignAxisB=+Z  SphDefPosRotationSequenceAxes=FollowerAxes  SphDefPosRotationSequence=XYX  SphDefPosRotationSequenceAngles=[0 0 0]  SphDefPosRotationSequenceAnglesUnits=deg  SphDefPosRotationMatrix=[1 0 0; 0 1 0; 0 0 1]  SphEqPosRotationMethod=None  SphEqPosRotationAngleUnits=deg  SphEqPosRotationStandardAxis=+Z  SphEqPosRotationAngle=0.0  SphEqPosRotationArbitraryAxis=[0 0 1]  SphEqPosFollAlignAxisA=+X  SphEqPosBaseAlignAxisA=+Y  SphEqPosFollAlignAxisB=+Y  SphEqPosBaseAlignAxisB=+Z  SphEqPosRotationSequenceAxes=FollowerAxes  SphEqPosRotationSequence=XYX  SphEqPosRotationSequenceAngles=[0 0 0]  SphEqPosRotationSequenceAnglesUnits=deg  SphEqPosRotationMatrix=[1 0 0; 0 1 0; 0 0 1]  SphSpringStiffness=0  SphSpringStiffnessUnits=N*m/deg  SphDampingCoefficient=0  SphDampingCoefficientUnits=N*m/(deg/s)  SphActuateTorqueX=off  SphActuateTorqueY=off  SphActuateTorqueZ=off  SphActuateTorque=off  SphTorqueActuationMode=NoTorque  SphMotionActuationMode=ComputedMotion  SphActuationFrame=BaseFrame  SphSensePosition=off  SphSenseVelocityX=off  SphSenseVelocityY=off  SphSenseVelocityZ=off  SphSenseVelocity=off  SphSenseAccelerationX=off  SphSenseAccelerationY=off  SphSenseAccelerationZ=off  SphSenseAcceleration=off  SphSenseTorqueX=off  SphSenseTorqueY=off  SphSenseTorqueZ=off  SphSenseTorqueForce=off  SphSenseLowerLimitTorqueMag=off  SphSenseUpperLimitTorqueMag=off  SphSensingFrame=BaseFrame  SphLowerLimitSpecify=off  SphLowerLimitBound=15  SphLowerLimitBoundUnits=deg  SphLowerLimitStiffness=1e4  SphLowerLimitStiffnessUnits=N*m/deg  SphLowerLimitDamping=10  SphLowerLimitDampingUnits=N*m/(deg/s)  SphLowerLimitTransitionRegionWidth=0.1  SphLowerLimitTransitionRegionWidthUnits=deg  SphUpperLimitSpecify=off  SphUpperLimitBound=45  SphUpperLimitBoundUnits=deg  SphUpperLimitStiffness=1e4  SphUpperLimitStiffnessUnits=N*m/deg  SphUpperLimitDamping=10  SphUpperLimitDampingUnits=N*m/(deg/s)  SphUpperLimitTransitionRegionWidth=0.1  SphUpperLimitTransitionRegionWidthUnits=deg  SphPositionTargetRotationMethod=None  SphPositionTargetRotationAngleUnits=deg  SphPositionTargetRotationStandardAxis=+Z  SphPositionTargetRotationAngle=0.0  SphPositionTargetRotationArbitraryAxis=[0 0 1]  SphPositionTargetFollAlignAxisA=+X  SphPositionTargetBaseAlignAxisA=+Y  SphPositionTargetFollAlignAxisB=+Y  SphPositionTargetBaseAlignAxisB=+Z  SphPositionTargetRotationSequenceAxes=FollowerAxes  SphPositionTargetRotationSequence=XYX  SphPositionTargetRotationSequenceAngles=[0 0 0]  SphPositionTargetRotationSequenceAnglesUnits=deg  SphPositionTargetRotationMatrix=[1 0 0; 0 1 0; 0 0 1]  SphPositionTargetSpecify=off  SphPositionTargetPriority=High  SphVelocityTargetValue=[0 0 0]  SphVelocityTargetValueUnits=deg/s  SphVelocityTargetSpecify=off  SphVelocityTargetPriority=High  SphVelocityTargetInFollowerFrame=on
  Body_Frame_2_RIGID : Subsystem
  Clock : Clock
  Leg_Assembly_1 : Subsystem
  Leg_Assembly_2 : Subsystem
  Leg_Assembly_3 : Subsystem
  "Leg_Assembly_4 " : Subsystem
  MechanismConfiguration : sm_lib/Utilities/Mechanism Configuration  UniformGravity=Constant  GravityVector=[0 -9.80665 0]  GravityUnits=m/s^2  LinearizationDelta=0.001
  Mux : Mux
  Mux{1..5} (5 alike) : Mux  Inputs=3
  PS-Simulink Converter{,1..5,7..15} (15 alike) : nesl_utility/PS-Simulink Converter  PhysicalDomain=network_engine_domain  SubClassName=ps_output  LeftPortType=input  RightPortType=output  PseudoPeriodic=off  Frequencies=[]  Unit=mm  AffineConversion=off
  "Scope " : Scope  NumInputPorts=3
  Scope 3 : Scope  NumInputPorts=4
  Simulink-PS Convert1 : nesl_utility/Simulink-PS Converter  PhysicalDomain=network_engine_domain  SubClassName=ps_input  LeftPortType=input  RightPortType=output  PseudoPeriodic=off  Frequencies=[]  NoiseDistribution=none  NoiseParameters=[]  Unit=1  AffineConversion=off  FilteringAndDerivatives=filter  SimscapeFilterOrder=2  InputFilterTimeConstant=0.001  UdotUserProvided=0
  Simulink-PS Converter{,2..7} (7 alike) : nesl_utility/Simulink-PS Converter  PhysicalDomain=network_engine_domain  SubClassName=ps_input  LeftPortType=input  RightPortType=output  PseudoPeriodic=off  Frequencies=[]  NoiseDistribution=none  NoiseParameters=[]  Unit=1  AffineConversion=off  FilteringAndDerivatives=filter  SimscapeFilterOrder=2  InputFilterTimeConstant=0.001  UdotUserProvided=0
  Solver Configuration : nesl_utility/Solver Configuration  PhysicalDomain=network_engine_domain  SubClassName=solver  LeftPortType=input  RightPortType=generic  Tones=[]  Harmonics=[]  SimulateNoise=off  Profile=off  UseLocalSampling=off  EnableSwitchedLinearOptims=on  FrequencyDomain=off  UseCCode=off  RelTol=0.001  AbsTol=1e-06  MinStep=1e-09  ToWorkspace=off  RevertToSquareIcSolve=off  NumHomotopyIterations=100  PhasorMode=off  PhasorModeNumHarmonics=1  DoDC=off  ResidualTolerance=1e-8  UseLocalSolver=off  LocalSolverChoice=NE_BACKWARD_EULER_ADVANCER  LocalSolverSampleTime=0.001  DoFixedCost=off  MaxNonlinIter=3  MaxModeIter=2  LinearAlgebra=Full  EquationFormulation=NE_TIME_EF  DelaysMemoryBudget=1024  AutomaticFiltering=on  FilteringTimeConstant=0.001  PartitionStorageMethod=AS_NEEDED  PartitionMemoryBudget=1024  PartitionMethod=ROBUST
  Sphere to Plane Force{,1..3} (4 alike) : Contact_Forces_Lib/3D/Sphere to Plane Force  sphere_rad=Sphere_R_1  plane_lenx=Plane_x  plane_leny=Plane_y  plane_depth=Plane_d  force_law=Linear  k_contact=Contact_Stiff_1  b_contact=Contact_Damp_1  pen_full_damp_F=1e-4  pen_exponent=1  custom_param_1=1  custom_param_2=1  friction_law=Stick-Slip Continuous  mu_kinetic=Coff_KF_1  mu_static=Coff_SF_1  v_thr=Thres_Vel_1  vis_on=off  vis_opc_en=0  vis_len_plaBz=0.005  vis_clr=[0.9 0.2 0.2]  vis_opc=0.7
  Sphere to Plane Force{4..9} (6 alike) : Contact_Forces_Lib/3D/Sphere to Plane Force  sphere_rad=Sphere_R_2  plane_lenx=Plane_x  plane_leny=Plane_y  plane_depth=Plane_d  force_law=Linear  k_contact=Contact_Stiff_2  b_contact=Contact_Damp_2  pen_full_damp_F=1e-4  pen_exponent=1  custom_param_1=1  custom_param_2=1  friction_law=Stick-Slip Continuous  mu_kinetic=Coff_KF_2  mu_static=Coff_SF_2  v_thr=Thres_Vel_2  vis_on=off  vis_opc_en=0  vis_len_plaBz=0.005  vis_clr=[0.9 0.2 0.2]  vis_opc=0.7
  To Workspace : ToWorkspace  VariableName=simout  SaveFormat=Timeseries  SampleTime=-1
  To Workspace1 : ToWorkspace  VariableName=simout1  SaveFormat=Timeseries  SampleTime=-1
  Transform : sm_lib/Frames and Transforms/Rigid Transform  TranslationMethod=Cartesian  TranslationStandardOffset=0  TranslationLengthUnit=mm  TranslationStandardAxis=+Z  TranslationCartesianOffset=smiData.RigidTransform(33).translation  TranslationROffset=0  TranslationROffsetUnits=m  TranslationZOffset=0  TranslationZOffsetUnits=m  TranslationThetaOffset=0  TranslationThetaOffsetUnits=deg  RotationMethod=ArbitraryAxis  RotationAngleUnits=rad  RotationStandardAxis=+Z  RotationAngle=smiData.RigidTransform(33).angle  RotationArbitraryAxis=smiData.RigidTransform(33).axis  FollAlignAxisA=+X  BaseAlignAxisA=+Y  FollAlignAxisB=+Y  BaseAlignAxisB=+Z  RotationSequenceAxes=FollowerAxes  RotationSequence=XYX  RotationSequenceAngles=[0 0 0]  RotationSequenceAnglesUnits=deg  RotationMatrix=[1 0 0; 0 1 0; 0 0 1]
  Transform Sensor : sm_lib/Frames and Transforms/Transform Sensor  MeasurementFrame=World  SenseAngle=off  SenseAxis=off  SenseAngle1=off  SenseAngle2=off  SenseAngle3=off  SenseQ=off  SenseR=off  SenseOmegaX=off  SenseOmegaY=off  SenseOmegaZ=off  SenseOmega1=off  SenseOmega2=off  SenseOmega3=off  SenseQDot=off  SenseRDot=off  SenseAlphaX=off  SenseAlphaY=off  SenseAlphaZ=off  SenseAlpha1=off  SenseAlpha2=off  SenseAlpha3=off  SenseQDDot=off  SenseRDDot=off  SenseX=on  SenseY=on  SenseZ=on  SenseRad=off  SenseAzim=off  SenseDist=off  SenseInc=off  SenseXDot=on  SenseYDot=off  SenseZDot=off  SenseRadDot=off  SenseAzimDot=off  SenseDistDot=off  SenseIncDot=off  SenseXDDot=off  SenseYDDot=off  SenseZDDot=off  SenseRadDDot=off  SenseAzimDDot=off  SenseDistDDot=off  SenseIncDDot=off
  Transform Sensor{1..4} (4 alike) : sm_lib/Frames and Transforms/Transform Sensor  MeasurementFrame=Base  SenseAngle=off  SenseAxis=off  SenseAngle1=off  SenseAngle2=off  SenseAngle3=off  SenseQ=off  SenseR=off  SenseOmegaX=off  SenseOmegaY=off  SenseOmegaZ=off  SenseOmega1=off  SenseOmega2=off  SenseOmega3=off  SenseQDot=off  SenseRDot=off  SenseAlphaX=off  SenseAlphaY=off  SenseAlphaZ=off  SenseAlpha1=off  SenseAlpha2=off  SenseAlpha3=off  SenseQDDot=off  SenseRDDot=off  SenseX=on  SenseY=on  SenseZ=on  SenseRad=off  SenseAzim=off  SenseDist=off  SenseInc=off  SenseXDot=off  SenseYDot=off  SenseZDot=off  SenseRadDot=off  SenseAzimDot=off  SenseDistDot=off  SenseIncDot=off  SenseXDDot=off  SenseYDDot=off  SenseZDDot=off  SenseRadDDot=off  SenseAzimDDot=off  SenseDistDDot=off  SenseIncDDot=off
  Transform1 : sm_lib/Frames and Transforms/Rigid Transform  TranslationMethod=Cartesian  TranslationStandardOffset=0  TranslationLengthUnit=mm  TranslationStandardAxis=+Z  TranslationCartesianOffset=smiData.RigidTransform(34).translation  TranslationROffset=0  TranslationROffsetUnits=m  TranslationZOffset=0  TranslationZOffsetUnits=m  TranslationThetaOffset=0  TranslationThetaOffsetUnits=deg  RotationMethod=ArbitraryAxis  RotationAngleUnits=rad  RotationStandardAxis=+Z  RotationAngle=smiData.RigidTransform(34).angle  RotationArbitraryAxis=smiData.RigidTransform(34).axis  FollAlignAxisA=+X  BaseAlignAxisA=+Y  FollAlignAxisB=+Y  BaseAlignAxisB=+Z  RotationSequenceAxes=FollowerAxes  RotationSequence=XYX  RotationSequenceAngles=[0 0 0]  RotationSequenceAnglesUnits=deg  RotationMatrix=[1 0 0; 0 1 0; 0 0 1]
  Weld Joint : sm_lib/Joints/Weld Joint  JointMode=Normal  SenseConstraintForce=off  SenseConstraintForceX=off  SenseConstraintForceY=off  SenseConstraintForceZ=off  SenseConstraintTorque=off  SenseConstraintTorqueX=off  SenseConstraintTorqueY=off  SenseConstraintTorqueZ=off  SenseTotalForce=off  SenseTotalForceX=off  SenseTotalForceY=off  SenseTotalForceZ=off  SenseTotalTorque=off  SenseTotalTorqueX=off  SenseTotalTorqueY=off  SenseTotalTorqueZ=off  CompositeWrenchDir=FollowerOnBase  CompositeWrenchFrame=BaseFrame
  World : sm_lib/Frames and Transforms/World Frame
  cover_2_RIGID : Subsystem
  cover_IMU_1_RIGID : Subsystem
  floor_1_RIGID : Subsystem
  Sine Wave : Sin  IOType=siggen  SampleTime=0
  wires:
  4Leg_Motion/4(theta_2_2) -> Simulink-PS Convert1/1
  4Leg_Motion/2(theta_1_2) -> Simulink-PS Converter3/1
  4Leg_Motion/6(theta_3_2) -> Simulink-PS Converter7/1
  4Leg_Motion/3(theta_2_1) -> Simulink-PS Converter/1
  4Leg_Motion/7(theta_4_1) -> Simulink-PS Converter4/1
  4Leg_Motion/8(theta_4_2) -> Simulink-PS Converter5/1
  4Leg_Motion/1(theta_1_1) -> Simulink-PS Converter2/1
  4Leg_Motion/5(theta_3_1) -> Simulink-PS Converter6/1
  Clock/1 -> 4Leg_Motion/1(time)
  PS-Simulink Converter3/1 -> Mux4/1
  PS-Simulink Converter5/1 -> Mux4/3
  PS-Simulink Converter4/1 -> Mux4/2
  PS-Simulink Converter/1 -> Mux5/1, "Scope "/1
  PS-Simulink Converter1/1 -> Mux5/2, "Scope "/2
  PS-Simulink Converter2/1 -> Mux5/3, "Scope "/3
  Sphere to Plane Force1/1 -> Scope 3/1
  PS-Simulink Converter9/1 -> Mux3/3
  PS-Simulink Converter7/1 -> Mux3/1
  PS-Simulink Converter8/1 -> Mux3/2
  PS-Simulink Converter12/1 -> Mux2/3
  PS-Simulink Converter10/1 -> Mux2/1
  PS-Simulink Converter11/1 -> Mux2/2
  PS-Simulink Converter15/1 -> Mux1/3
  PS-Simulink Converter13/1 -> Mux1/1
  PS-Simulink Converter14/1 -> Mux1/2
  Mux/1 -> To Workspace/1
  Mux4/1 -> Mux/4
  Mux3/1 -> Mux/3
  Mux2/1 -> Mux/2
  Mux1/1 -> Mux/1
  Mux5/1 -> To Workspace1/1
  connections:
  Transform/LConn1 -- Transform1/LConn1 -- Solver Configuration/RConn1 -- MechanismConfiguration/RConn1 -- World/RConn1
  Body_Frame_2_RIGID/LConn6 -- cover_IMU_1_RIGID/LConn1
  Body_Frame_2_RIGID/LConn5 -- Leg_Assembly_3/LConn1
  Body_Frame_2_RIGID/LConn4 -- "Leg_Assembly_4 "/LConn1
  Body_Frame_2_RIGID/LConn3 -- Leg_Assembly_1/LConn1
  Body_Frame_2_RIGID/LConn2 -- Leg_Assembly_2/LConn1
  Body_Frame_2_RIGID/LConn1 -- cover_2_RIGID/LConn2
  cover_2_RIGID/LConn1 -- 6-DOF Joint1/RConn1
  6-DOF Joint1/LConn1 -- Transform1/RConn1
  Sphere to Plane Force/LConn1 -- Leg_Assembly_2/RConn1
  Sphere to Plane Force9/RConn1 -- Sphere to Plane Force8/RConn1 -- Sphere to Plane Force7/RConn1 -- Sphere to Plane Force6/RConn1 -- Sphere to Plane Force5/RConn1 -- Sphere to Plane Force4/RConn1 -- Sphere to Plane Force2/RConn1 -- Sphere to Plane Force3/RConn1 -- Sphere to Plane Force1/RConn1 -- Sphere to Plane Force/RConn1 -- floor_1_RIGID/LConn2
  Transform/RConn1 -- Weld Joint/LConn1
  Weld Joint/RConn1 -- floor_1_RIGID/LConn1
  Sphere to Plane Force2/LConn1 -- "Leg_Assembly_4 "/RConn1
  Sphere to Plane Force3/LConn1 -- Leg_Assembly_3/RConn1
  Sphere to Plane Force1/LConn1 -- Leg_Assembly_1/RConn1
  Simulink-PS Converter/RConn1 -- Leg_Assembly_2/LConn2
  Simulink-PS Convert1/RConn1 -- Leg_Assembly_2/LConn3
  Sphere to Plane Force4/LConn1 -- cover_2_RIGID/LConn3
  Sphere to Plane Force5/LConn1 -- cover_2_RIGID/LConn4
  Sphere to Plane Force6/LConn1 -- cover_2_RIGID/LConn5
  Sphere to Plane Force7/LConn1 -- cover_2_RIGID/LConn6
  Sphere to Plane Force8/LConn1 -- cover_2_RIGID/LConn7
  Sphere to Plane Force9/LConn1 -- cover_2_RIGID/LConn8
  Simulink-PS Converter3/RConn1 -- Leg_Assembly_1/LConn3
  Simulink-PS Converter2/RConn1 -- Leg_Assembly_1/LConn2
  Simulink-PS Converter4/RConn1 -- "Leg_Assembly_4 "/LConn2
  Simulink-PS Converter5/RConn1 -- "Leg_Assembly_4 "/LConn3
  Simulink-PS Converter6/RConn1 -- Leg_Assembly_3/LConn2
  Simulink-PS Converter7/RConn1 -- Leg_Assembly_3/LConn3
  Transform Sensor/RConn1 -- Transform Sensor4/LConn1 -- Transform Sensor3/LConn1 -- Transform Sensor2/LConn1 -- Transform Sensor1/LConn1 -- Body_Frame_2_RIGID/LConn7
  Transform Sensor1/RConn4 -- PS-Simulink Converter5/LConn1
  Transform Sensor1/RConn2 -- PS-Simulink Converter3/LConn1
  Transform Sensor1/RConn3 -- PS-Simulink Converter4/LConn1
  Transform Sensor1/RConn1 -- Leg_Assembly_1/RConn2
  Transform Sensor/RConn3 -- PS-Simulink Converter/LConn1
  Transform Sensor/RConn4 -- PS-Simulink Converter1/LConn1
  Transform Sensor2/RConn1 -- Leg_Assembly_2/RConn2
  Transform Sensor2/RConn2 -- PS-Simulink Converter7/LConn1
  Transform Sensor2/RConn3 -- PS-Simulink Converter8/LConn1
  Transform Sensor2/RConn4 -- PS-Simulink Converter9/LConn1
  Transform Sensor3/RConn1 -- Leg_Assembly_3/RConn2
  Transform Sensor3/RConn2 -- PS-Simulink Converter10/LConn1
  Transform Sensor3/RConn3 -- PS-Simulink Converter11/LConn1
  Transform Sensor3/RConn4 -- PS-Simulink Converter12/LConn1
  Transform Sensor4/RConn1 -- "Leg_Assembly_4 "/RConn2
  Transform Sensor4/RConn2 -- PS-Simulink Converter13/LConn1
  Transform Sensor4/RConn3 -- PS-Simulink Converter14/LConn1
  Transform Sensor4/RConn4 -- PS-Simulink Converter15/LConn1
  Transform Sensor/RConn2 -- PS-Simulink Converter2/LConn1
